simulink library "commblksprivate"  (Simulink 6.0)
libraries: dspsigattribs x2, dspswit3 x1, simulink_extras x1, dspmathops x1
settings Model: CovMetricSettings=d  Creator=mshakeri  LastModifiedBy=akansal  ExtModeAutoUpdateStatusClock=off  ProdHWDeviceType=Specified
settings Model: ForwardingTableString=|
  | ||__slOldName__||commblksprivate/3-stage
  | Decimator||__slNewName__||cbobsv2p5/3-stage
  | Decimator||__slOldName__||commblksprivate/FSK//CPM
  | Frequency
  | Down-Converter||__slNewName__||cbobsv2p5/FSK//CPM
  | Frequency
  | Down-Converter||__slOldName__||commblksprivate/PAM//QAM//PSK
  | Frequency
  | Down-Converter||__slNewName__||cbobsv2p5/PAM//QAM//PSK
  | Frequency
  | Down-Converter||__slOldName__||commblksprivate/3-stage
  | Interpolator||__slNewName__||cbobsv2p5/3-stage
  | Interpolator||__slOldName__||commblksprivate/FSK//CPM
  | Frequency
  | Up-Converter||__slNewName__||cbobsv2p5/FSK//CPM
  | Frequency
  | Up-Converter||__slOldName__||commblksprivate/PAM//QAM//PSK
  | Frequency
  | Up-Converter||__slNewName__||cbobsv2p5/PAM//QAM//PSK
  | Frequency
  | Up-Converter||__slOldName__||commblksprivate/Frequency
  | Down-Converter||__slNewName__||cbobsv2p5/PAM//QAM//PSK
  | Frequency
  | Down-Converter||__slOldName__||commblksprivate/Frequency
  | Up-Converter||__slNewName__||cbobsv2p5/PAM//QAM//PSK
  | Frequency
  | Up-Converter

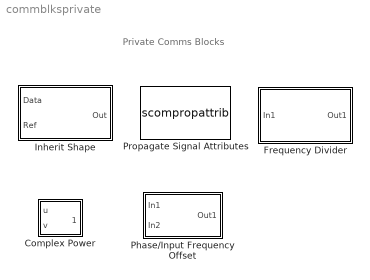
== system commblksprivate ==
  note: Private Comms Blocks
  Complex Power : Subsystem
      mask Type: Complex Power
      mask Description: Raise the input U to the power V.
  Frequency Divider : Subsystem  mask(Frequency Divider){n=2}
      mask prompts: n "Divide frequency by"
      mask help: Divide frequency of input square wave by an integer.
      mask Help: Enter an integer by which you want to divide the input frequency.
      mask Display: disp(['Divide Frequency\nby ' get_param(gcb, 'n')])
  Inherit Shape : Subsystem
      mask Type: Inherit Shape
      mask Description: Reshape Data input signal using the Reference signal. Output signal has the same number of elements as Data input, and has the same shape as Reference input.
      mask Display: text(.9,0.5,'Inherit\nShape','horiz','right');
  Phase/Input Frequency Offset : Subsystem  mask(Phase/Input Frequency Offset){phaseOffset=0}
      mask prompts: phaseOffset "Phase offset (deg):"
      mask help: Complex baseband model of residual phase and input frequency offsets.
      mask Display: disp('Phase/\nInput Freq\nOffset');
  Propagate Signal Attributes : S-Function  FunctionName=scompropattrib
      mask Type: Propagate signal attributes
      mask Description: Propagate signal dimensions, sample time and complexity from port 1 to port 2.
      mask Display: disp('Propagate Signal\n Attributes')

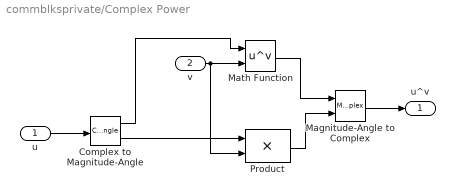
== system commblksprivate/Complex Power ==
  u : Inport
  v : Inport  Port=2
  Complex to Magnitude-Angle : ComplexToMagnitudeAngle
  Magnitude-Angle to Complex : MagnitudeAngleToComplex
  Math Function : Math  Operator=pow  OutputSignalType=real  SaturateOnIntegerOverflow=on
  Product : Product  SaturateOnIntegerOverflow=on  InputSameDT=on
  u^v : Outport
  wires:
  Magnitude-Angle to Complex/1 -> u^v/1
  Product/1 -> Magnitude-Angle to Complex/2
  Math Function/1 -> Magnitude-Angle to Complex/1
  u/1 -> Complex to Magnitude-Angle/1
  v/1 -> Math Function/2, Product/2
  Complex to Magnitude-Angle/1 -> Math Function/1
  Complex to Magnitude-Angle/2 -> Product/1

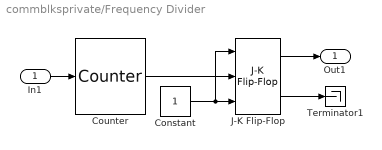
== system commblksprivate/Frequency Divider ==
  In1 : Inport
  Constant : Constant
  Counter : dspswit3/Counter  Direction=Up  CountEvent=Either edge  CounterSize=User defined  MaxCount=n-1  InitialCount=0  Output=Hit  HitValue=n-1  ResetInput=off  SamplesPerFrame=1  Ts=1
  J-K Flip-Flop : simulink_extras/Flip Flops/J-K Flip-Flop  initial_condition=0
  Terminator1 : Terminator
  Out1 : Outport
  wires:
  J-K Flip-Flop/2 -> Terminator1/1
  Constant/1 -> J-K Flip-Flop/1, J-K Flip-Flop/3
  Counter/1 -> J-K Flip-Flop/2
  J-K Flip-Flop/1 -> Out1/1
  In1/1 -> Counter/1

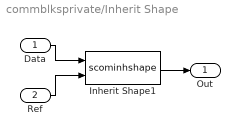
== system commblksprivate/Inherit Shape ==
  Data : Inport
  Ref : Inport  Port=2
  Inherit Shape1 : S-Function  FunctionName=scominhshape
  Out : Outport
  wires:
  Inherit Shape1/1 -> Out/1
  Data/1 -> Inherit Shape1/1
  Ref/1 -> Inherit Shape1/2

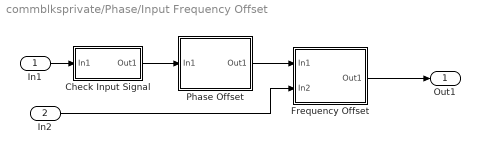
== system commblksprivate/Phase/Input Frequency Offset ==
  In1 : Inport
  In2 : Inport  Port=2
  Check Input Signal : Subsystem
      mask Display: disp('Check\nInput Signal');
  Frequency Offset : Subsystem
      mask Display: disp('Frequency\nOffset');
  Phase Offset : Subsystem
      mask Display: disp('Phase\nOffset');
  Out1 : Outport
  wires:
  In2/1 -> Frequency Offset/2(In2)
  Frequency Offset/1(Out1) -> Out1/1
  In1/1 -> Check Input Signal/1(In1)
  Phase Offset/1(Out1) -> Frequency Offset/1(In1)
  Check Input Signal/1(Out1) -> Phase Offset/1(In1)

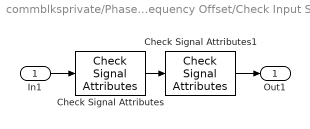
== system commblksprivate/Phase/Input Frequency Offset/Check Input Signal ==
  In1 : Inport
  Check Signal Attributes : dspsigattribs/Check Signal Attributes  SigAttribCheckMethod=Does not match attributes exactly  Complexity=Complex  Frame=Ignore  DimsCheckMethod=Is...  Dimensions=Column vector (2-D) or scalar  DatatypeCheckMethod=Ignore  DatatypeGeneral=Boolean  DtypeFloatSpecific=Any floating-point  DtypeFixedSpecific=Any fixed-point  DtypeIntSpecific=Any integer  SampleMode=Ignore
  Check Signal Attributes1 : dspsigattribs/Check Signal Attributes  SigAttribCheckMethod=Matches attributes exactly  Complexity=Ignore  Frame=Sample-based  DimsCheckMethod=Is...  Dimensions=Vector (1-D or 2-D)  DatatypeCheckMethod=Ignore  DatatypeGeneral=Boolean  DtypeFloatSpecific=Any floating-point  DtypeFixedSpecific=Any fixed-point  DtypeIntSpecific=Any integer  SampleMode=Ignore
  Out1 : Outport
  wires:
  Check Signal Attributes/1 -> Check Signal Attributes1/1
  Check Signal Attributes1/1 -> Out1/1
  In1/1 -> Check Signal Attributes/1

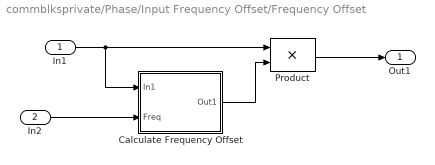
== system commblksprivate/Phase/Input Frequency Offset/Frequency Offset ==
  In1 : Inport
  In2 : Inport  Port=2
  Calculate Frequency Offset : Subsystem
      mask Display: disp('Calculate\nFrequency\nOffset');
  Product : Product  SaturateOnIntegerOverflow=on  InputSameDT=on
  Out1 : Outport
  wires:
  In2/1 -> Calculate Frequency Offset/2(Freq)
  Product/1 -> Out1/1
  In1/1 -> Calculate Frequency Offset/1(In1), Product/1
  Calculate Frequency Offset/1(Out1) -> Product/2

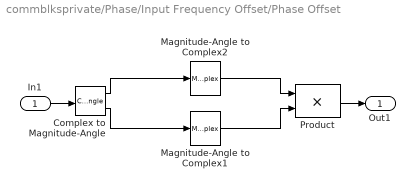
== system commblksprivate/Phase/Input Frequency Offset/Phase Offset ==
  In1 : Inport
  Complex to Magnitude-Angle : ComplexToMagnitudeAngle
  Magnitude-Angle to Complex1 : MagnitudeAngleToComplex  Input=Angle  ConstantPart=1
  Magnitude-Angle to Complex2 : MagnitudeAngleToComplex  Input=Magnitude  ConstantPart=phaseOffset*pi/180
  Product : Product  SaturateOnIntegerOverflow=on  InputSameDT=on
  Out1 : Outport
  wires:
  Complex to Magnitude-Angle/2 -> Magnitude-Angle to Complex1/1
  Complex to Magnitude-Angle/1 -> Magnitude-Angle to Complex2/1
  Magnitude-Angle to Complex2/1 -> Product/1
  Magnitude-Angle to Complex1/1 -> Product/2
  In1/1 -> Complex to Magnitude-Angle/1
  Product/1 -> Out1/1

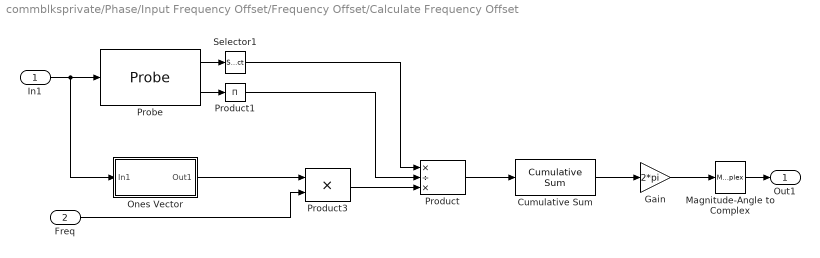
== system commblksprivate/Phase/Input Frequency Offset/Frequency Offset/Calculate Frequency Offset ==
  In1 : Inport
  Freq : Inport  Port=2
  Cumulative Sum : dspmathops/Cumulative Sum  dim=Channels (running sum)  reset_popup=None
  Gain : Gain  Gain=2*pi  SaturateOnIntegerOverflow=on
  Magnitude-Angle to Complex : MagnitudeAngleToComplex  Input=Angle  ConstantPart=1
  Ones Vector : Subsystem
      mask Type: Ones Vector
      mask Description: Create a vector of equals whose length is equal to input portwidth.
      mask Display: disp('Ones(1:length)')
  Probe : Probe  ProbeWidth=off  ProbeComplexSignal=off  ProbeSignalDimensions=on
  Product : Product  Inputs=*/*  SaturateOnIntegerOverflow=on  InputSameDT=on
  Product1 : Product  Inputs=1  SaturateOnIntegerOverflow=on  InputSameDT=on
  Product3 : Product  Inputs=**  SaturateOnIntegerOverflow=on
  Selector1 : Selector  Elements=[1 ]  InputPortWidth=2
  Out1 : Outport
  wires:
  Selector1/1 -> Product/1
  Product1/1 -> Product/2
  Probe/1 -> Selector1/1
  Product/1 -> Cumulative Sum/1
  Probe/2 -> Product1/1
  In1/1 -> Probe/1, Ones Vector/1(In1)
  Magnitude-Angle to Complex/1 -> Out1/1
  Gain/1 -> Magnitude-Angle to Complex/1
  Product3/1 -> Product/3
  Freq/1 -> Product3/2
  Cumulative Sum/1 -> Gain/1
  Ones Vector/1(Out1) -> Product3/1

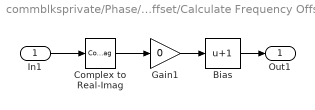
== system commblksprivate/Phase/Input Frequency Offset/Frequency Offset/Calculate Frequency Offset/Ones Vector ==
  In1 : Inport
  Bias : Bias  Bias=1
  Complex to Real-Imag : ComplexToRealImag  Output=Real
  Gain1 : Gain  Gain=0
  Out1 : Outport
  wires:
  Complex to Real-Imag/1 -> Gain1/1
  Gain1/1 -> Bias/1
  In1/1 -> Complex to Real-Imag/1
  Bias/1 -> Out1/1
